simulink model "host_DSP_controller"  (R2018a)
settings: Solver=FixedStepDiscrete  StartTime=0  StopTime=Inf  RelTol=1e-6  EnableMultiTasking=on
undefined symbols (not defined in the file): i
libraries: powerlib x33, c2000scilib x3
settings Model: ExtModeTrigDuration=8  Creator=ENG.Ihab  LastModifiedBy=ihab
settings DataIOCC: LimitDataPoints=on  SaveFormat=Array  SignalLoggingSaveFormat=ModelDataLogs  SaveOutput=off  SaveTime=off
settings OptimizationCC: DefaultUnderspecifiedDataType=single  ExpressionDepthLimit=2147483647  LifeSpan=1  MaxStackSize=512
settings DebuggingCC: AlgebraicLoopMsg=none  UnderspecifiedInitializationDetection=Classic  MergeDetectMultiDrivingBlocksExec=none  FcnCallInpInsideContextMsg=warning  UnconnectedInputMsg=none  UnconnectedOutputMsg=none  UnconnectedLineMsg=none  StateNameClashWarn=warning  SFUnexpectedBacktrackingDiag=warning  SFNoUnconditionalDefaultTransitionDiag=warning  SFExecutionAtInitializationDiag=none
settings HardwareCC: ProdBitPerChar=16  ProdBitPerInt=16  ProdBitPerPointer=32  ProdBitPerSizeT=32  ProdBitPerPtrDiffT=32  ProdLargestAtomicInteger=Integer  ProdLargestAtomicFloat=None  ProdWordSize=16  ProdLongLongMode=on  ProdHWDeviceType=Texas Instruments->C2000  TargetBitPerChar=16  TargetBitPerInt=16  TargetLargestAtomicInteger=Integer  TargetIntDivRoundTo=Zero  TargetEndianess=LittleEndian  TargetWordSize=16  TargetHWDeviceType=Texas Instruments->C2000  ProdEqTarget=off
settings ModelReferenceCC: PropagateSignalLabelsOutOfModel=off
settings SFSimCC: SimParseCustomCode=off  MATLABDynamicMemAlloc=off
settings RTWCC: SystemTargetFile=ert.tlc  HardwareBoard=TI F281x  TLCOptions=-aInlineSetEventsForThisBaseRateFcn=TLC_FALSE -aSuppressMultiTaskScheduler=TLC_FALSE -aRateBasedStepFcn=1  TemplateMakefile=ert_default_tmf  Toolchain=Texas Instruments Code Composer Studio (C2000)
settings CodeAppCC: IgnoreCustomStorageClasses=off  CustomSymbolStrType=$N$R$M  StateflowObjectComments=on  InternalIdentifier=Classic
settings ERTTargetCC: CodeReplacementLibrary=TI C28x  MultiwordLength=2048  ParMdlRefBuildCompliant=off  SupportComplex=off  CPPClassGenCompliant=off  ExtModeMexFile=TIC2000ExternalModeOpen  ExtModeIntrfLevel=Level2 - Open  ConvertIfToSwitch=off  SuppressUnreachableDefaultCases=off
settings ConfigComp: CovMetricSettings=dw  CovHtmlReporting=on  CovSaveCumulativeToWorkspaceVar=on  CovSaveSingleToWorkspaceVar=on  CovExternalEMLEnable=off
settings SimscapeCC: SimscapeNormalizeSystem=off

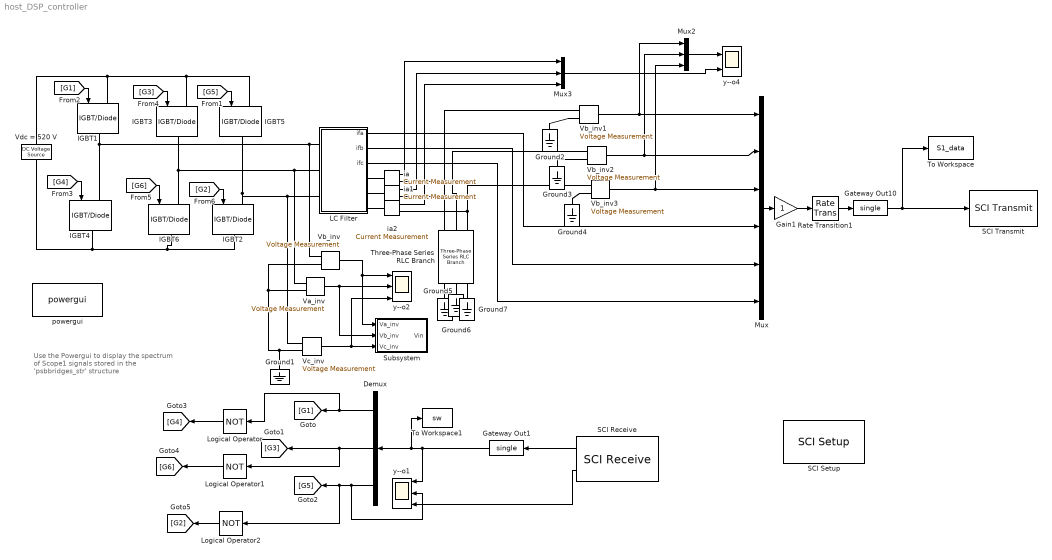
== system host_DSP_controller ==
  note: Use the Powergui to display
      | the spectrum of Scope1 signals
      | stored in the  'psbbridges_str'
      | structure
  Demux : Demux  Outputs=3
  Gain1 : Gain
  Gateway Out1 : DataTypeConversion  OutDataTypeStr=single  RndMeth=Simplest
  Gateway Out10 : DataTypeConversion  OutDataTypeStr=single  RndMeth=Nearest
  Ground{1..7} (7 alike) : powerlib/Elements/Ground  LConnTagsString=a
  IGBT{1..6} (6 alike) : powerlib/Power Electronics/IGBT//Diode  Ron=1e-3  Rs=1e5  Cs=inf  Measurements=off
  LC Filter : Subsystem
  Logical Operator : Logic  Operator=NOT  AllPortsSameDT=off  OutDataTypeStr=boolean
  Logical Operator1 : Logic  Operator=NOT  AllPortsSameDT=off  OutDataTypeStr=boolean
  Logical Operator2 : Logic  Operator=NOT  AllPortsSameDT=off  OutDataTypeStr=boolean
  Mux : Mux  Inputs=6
  Mux2 : Mux  Inputs=3
  Mux3 : Mux  Inputs=3
  Rate Transition1 : RateTransition  Integrity=off  OutPortSampleTime=2.2*70e-6
  SCI Receive : c2000scilib/SCI Receive  module=COM 1  dataHead='S'  dataTail='E'  dataType=single  dataDim=3  initValue=0  errOption=Output the last received value  errValue=0  sampleTime=70e-6  outputStatus=on
      settings: SourceProductName=MATLAB Coder  SourceProductBaseCode=ME
  SCI Setup : c2000scilib/SCI Setup  Priority=-99  commModeA=protocol  baudRateA=115200  charLenA=8  stopBitA=1  parityA=odd  timeoutA=2  commModeB=raw data  baudRateB=115200  charLenB=8  stopBitB=1  parityB=none  timeoutB=1.0  commModeC=raw data  baudRateC=115200  charLenC=8  stopBitC=1  parityC=none  timeoutC=2  commModeD=raw data  baudRateD=115200  charLenD=8  stopBitD=1  parityD=none  timeoutD=10
      settings: SourceProductName=MATLAB Coder  SourceProductBaseCode=ME
  SCI Transmit : c2000scilib/SCI Transmit  module=COM 1  header='S'  tail='E'
      settings: SourceProductName=MATLAB Coder  SourceProductBaseCode=ME
  Subsystem : Subsystem
  Three-Phase Series RLC Branch : powerlib/Elements/Three-Phase Series RLC Branch  LConnTagsString=A|B|C  RConnTagsString=A|B|C  BranchType=R  Resistance=20  Inductance=1e-3  Capacitance=40e-6  Measurements=None
  To Workspace : ToWorkspace  VariableName=S1_data  SampleTime=-1
  To Workspace1 : ToWorkspace  VariableName=sw  SampleTime=-1
  Va_inv : powerlib/Measurements/Voltage Measurement  Tag=PoWeRsYsTeMmEaSuReMeNt  PhasorSimulation=off  OutputType=Magnitude  PSBequivalent=0
  Vb_inv{,1..3} (4 alike) : powerlib/Measurements/Voltage Measurement  Tag=PoWeRsYsTeMmEaSuReMeNt  PhasorSimulation=off  OutputType=Magnitude  PSBequivalent=0
  Vc_inv : powerlib/Measurements/Voltage Measurement  Tag=PoWeRsYsTeMmEaSuReMeNt  PhasorSimulation=off  OutputType=Magnitude  PSBequivalent=0
  Vdc = 520 V : powerlib/Electrical Sources/DC Voltage Source  Description=source block  Amplitude=520  Measurements=None
      settings: AttributesFormatString=\n
  ia : powerlib/Measurements/Current Measurement  PhasorSimulation=off  OutputType=Complex  PSBequivalent=0
  ia1 : powerlib/Measurements/Current Measurement  PhasorSimulation=off  OutputType=Complex  PSBequivalent=0
  ia2 : powerlib/Measurements/Current Measurement  PhasorSimulation=off  OutputType=Complex  PSBequivalent=0
  powergui : powerlib/powergui  SimulationMode=Discrete  SampleTime=70e-6  frequency=60  Iterations=50  frequencyindice=0  Pbase=100e6  ErrMax=1e-4  UnitsV=kV  UnitsW=MW  buscounter=0  FunctionMessages=off  echomessages=off  EnableUseOfTLC=off  CurrentSourceSwitches=off  DisableSnubberDevices=off  DisableRonSwitches=off  DisableVfSwitches=off  DisplayEquations=off  SolverType=Tustin/Backward Euler (TBE)  Interpol=off  ExternalGateDelay=off  methode=off  Ts=0  x0status=blocks  SPID=off  SwTol=0  HookPort=off  RestoreLinks=warning  ResistiveCurrentMeasurement=off  Frange=[0:2:500]  Ylog=off  Xlog=on  ShowGrid=off  save=off  variable=ZData  structure=vo_output  ZoomFFT=off  StartTime=0.1-2/50  cycles=2  DisplayStyle=1  fundamental=50  FreqAxis=off  MaxFrequency=500  frequencyindicesteady=1  RmsSteady=1  display=off
  y--o1 : Scope  NumInputPorts=3
  y--o2 : Scope  NumInputPorts=3
  y--o4 : Scope  NumInputPorts=2
  wires:
  Vb_inv1/1 -> Mux2/1, Mux/1
  Vb_inv2/1 -> Mux2/2, Mux/2
  Vb_inv3/1 -> Mux2/3, Mux/3
  [G3] -> IGBT3/1
  [G6] -> IGBT6/1
  [G2] -> IGBT2/1
  [G5] -> IGBT5/1
  [G1] -> IGBT1/1
  Demux/1 -> Logical Operator/1, [G1]
  Demux/2 -> Logical Operator1/1, [G3]
  Demux/3 -> Logical Operator2/1, [G5], y--o1/2
  Mux/1 -> Gain1/1
  LC Filter/1(ifa) -> Mux/4
  LC Filter/2(ifb) -> Mux/5
  LC Filter/3(ifc) -> Mux/6
  [G4] -> IGBT4/1
  Logical Operator1/1 -> [G6]
  Logical Operator2/1 -> [G2]
  Vb_inv/1 -> y--o2/1, Subsystem/1(Va_inv)
  Va_inv/1 -> y--o2/2, Subsystem/2(Vb_inv)
  Vc_inv/1 -> y--o2/3, Subsystem/3(Vc_inv)
  SCI Receive/1 -> Gateway Out1/1
  Gateway Out1/1 -> y--o1/1, Demux/1, To Workspace1/1
  SCI Receive/2 -> y--o1/3
  Gain1/1 -> Rate Transition1/1
  Rate Transition1/1 -> Gateway Out10/1
  ia/1 -> Mux3/1
  ia1/1 -> Mux3/2
  ia2/1 -> Mux3/3
  Mux2/1 -> y--o4/1
  Mux3/1 -> y--o4/2
  Logical Operator/1 -> [G4]
  Gateway Out10/1 -> To Workspace/1, SCI Transmit/1
  connections:
  Vb_inv2/LConn2 -- Ground3/LConn1
  Vb_inv3/LConn2 -- Ground4/LConn1
  IGBT4/RConn1 -- Vdc = 520 V/LConn1 -- IGBT2/RConn1 -- IGBT6/RConn1
  IGBT6/LConn1 -- IGBT3/RConn1 -- LC Filter/LConn2 -- Va_inv/LConn1
  Ground7/LConn1 -- Three-Phase Series RLC Branch/LConn3
  Ground6/LConn1 -- Three-Phase Series RLC Branch/LConn2
  Ground5/LConn1 -- Three-Phase Series RLC Branch/LConn1
  Vb_inv2/LConn1 -- ia1/RConn1 -- Three-Phase Series RLC Branch/RConn2
  Three-Phase Series RLC Branch/RConn1 -- ia/RConn1 -- Vb_inv1/LConn1
  Vdc = 520 V/RConn1 -- IGBT5/LConn1 -- IGBT3/LConn1 -- IGBT1/LConn1
  IGBT5/RConn1 -- IGBT2/LConn1 -- LC Filter/LConn3 -- Vc_inv/LConn1
  IGBT4/LConn1 -- IGBT1/RConn1 -- LC Filter/LConn1 -- Vb_inv/LConn1
  Vb_inv/LConn2 -- Va_inv/LConn2 -- Vc_inv/LConn2 -- Ground1/LConn1
  Three-Phase Series RLC Branch/RConn3 -- ia2/RConn1 -- Vb_inv3/LConn1
  Vb_inv1/LConn2 -- Ground2/LConn1
  LC Filter/RConn1 -- ia/LConn1
  LC Filter/RConn2 -- ia1/LConn1
  LC Filter/RConn3 -- ia2/LConn1

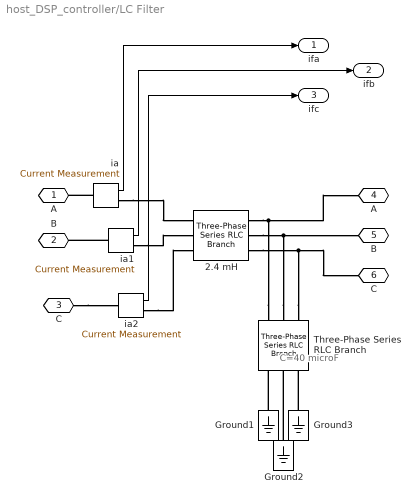
== system host_DSP_controller/LC Filter ==
  note: C=40 microF
  "2.4 mH " : powerlib/Elements/Three-Phase Series RLC Branch  LConnTagsString=A|B|C  RConnTagsString=A|B|C  BranchType=L  Resistance=1.0  Inductance=0.01  Capacitance=1.0  Measurements=None
  Ground1 : powerlib/Elements/Ground  LConnTagsString=a
  Ground2 : powerlib/Elements/Ground  LConnTagsString=a
  Ground3 : powerlib/Elements/Ground  LConnTagsString=a
  Three-Phase Series RLC Branch : powerlib/Elements/Three-Phase Series RLC Branch  LConnTagsString=A|B|C  RConnTagsString=A|B|C  BranchType=C  Resistance=1  Inductance=1e-3  Capacitance=500e-6  Measurements=None
  ia : powerlib/Measurements/Current Measurement  PhasorSimulation=off  OutputType=Complex  PSBequivalent=0
  ia1 : powerlib/Measurements/Current Measurement  PhasorSimulation=off  OutputType=Complex  PSBequivalent=0
  ia2 : powerlib/Measurements/Current Measurement  PhasorSimulation=off  OutputType=Complex  PSBequivalent=0
  A : PMIOPort  Side=Left
  B : PMIOPort  Port=2  Side=Left
  C : PMIOPort  Port=3  Side=Left
  "A " : PMIOPort  Port=4  Side=Right
  "B " : PMIOPort  Port=5  Side=Right
  "C " : PMIOPort  Port=6  Side=Right
  ifa : Outport
  ifb : Outport  Port=2
  ifc : Outport  Port=3
  wires:
  ia/1 -> ifa/1
  ia1/1 -> ifb/1
  ia2/1 -> ifc/1
  connections:
  Three-Phase Series RLC Branch/RConn1 -- "2.4 mH "/RConn1 -- "A "/RConn1
  Three-Phase Series RLC Branch/RConn2 -- "2.4 mH "/RConn2 -- "B "/RConn1
  Three-Phase Series RLC Branch/RConn3 -- "2.4 mH "/RConn3 -- "C "/RConn1
  ia/LConn1 -- A/RConn1
  ia/RConn1 -- "2.4 mH "/LConn1
  ia1/LConn1 -- B/RConn1
  C/RConn1 -- ia2/LConn1
  ia1/RConn1 -- "2.4 mH "/LConn2
  ia2/RConn1 -- "2.4 mH "/LConn3
  Ground1/LConn1 -- Three-Phase Series RLC Branch/LConn1
  Ground2/LConn1 -- Three-Phase Series RLC Branch/LConn2
  Ground3/LConn1 -- Three-Phase Series RLC Branch/LConn3

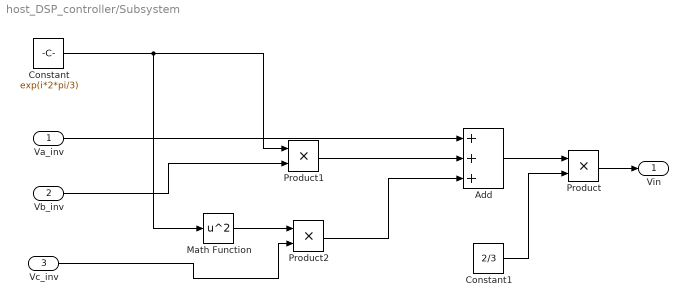
== system host_DSP_controller/Subsystem ==
  Va_inv : Inport
  Vb_inv : Inport  Port=2
  Vc_inv : Inport  Port=3
  Add : Sum  Inputs=+++
  Constant : Constant  Value=exp(i*2*pi/3)
  Constant1 : Constant  Value=2/3
  Math Function : Math  Operator=square  SaturateOnIntegerOverflow=on
  Product : Product  RndMeth=Zero
  Product1 : Product  RndMeth=Zero
  Product2 : Product  RndMeth=Zero
  Vin : Outport
  wires:
  Add/1 -> Product/1
  Va_inv/1 -> Add/1
  Constant1/1 -> Product/2
  Product1/1 -> Add/2
  Constant/1 -> Product1/1, Math Function/1
  Vb_inv/1 -> Product1/2
  Math Function/1 -> Product2/1
  Vc_inv/1 -> Product2/2
  Product2/1 -> Add/3
  Product/1 -> Vin/1
